simulink model "verify_Storage_Type_5_CONF_mdl"  (R2016b)
settings: Solver=ode45  StartTime=0  StopTime=6*3600  MaxStep=600  RelTol=1e-3  EnableMultiTasking=on
undefined symbols (not defined in the file or in its folder): path_carnot
libraries: carnot x20, simulink x6
settings Model: DEBUGGLOBALLEVEL=FATALLEVEL  DEBUGMAXTOTALWARNINGS=0  DEBUGMAXCONSECUTIVEWARNINGS=0  DEBUGWRITETOFILE=0  DEBUGFILENAME='error.txt'  Creator=drhf  LastModifiedBy=drhf
settings DataIOCC: SaveFormat=Array  SignalLoggingSaveFormat=ModelDataLogs
settings OptimizationCC: ExpressionDepthLimit=2147483647  LifeSpan=inf
settings DebuggingCC: UnderspecifiedInitializationDetection=Classic  MergeDetectMultiDrivingBlocksExec=none  SolverPrmCheckMsg=warning  FcnCallInpInsideContextMsg=warning  StateNameClashWarn=warning  SFUnexpectedBacktrackingDiag=warning  SFNoUnconditionalDefaultTransitionDiag=warning  SFExecutionAtInitializationDiag=none
settings HardwareCC: ProdBitPerPointer=32  ProdBitPerSizeT=32  ProdBitPerPtrDiffT=32  ProdLargestAtomicFloat=None  ProdIntDivRoundTo=Undefined  ProdEndianess=Unspecified  ProdWordSize=32  ProdHWDeviceType=32-bit Generic
settings ModelReferenceCC: PropagateSignalLabelsOutOfModel=off
settings GRTTargetCC: TargetLangStandard=C89/C90 (ANSI)  GeneratePreprocessorConditionals=Disable all  CombineOutputUpdateFcns=off  GRTInterface=on
settings ConfigComp: CovMetricSettings=dw  CovHtmlReporting=on  CovSaveCumulativeToWorkspaceVar=on  CovSaveSingleToWorkspaceVar=on  CovExternalEMLEnable=off

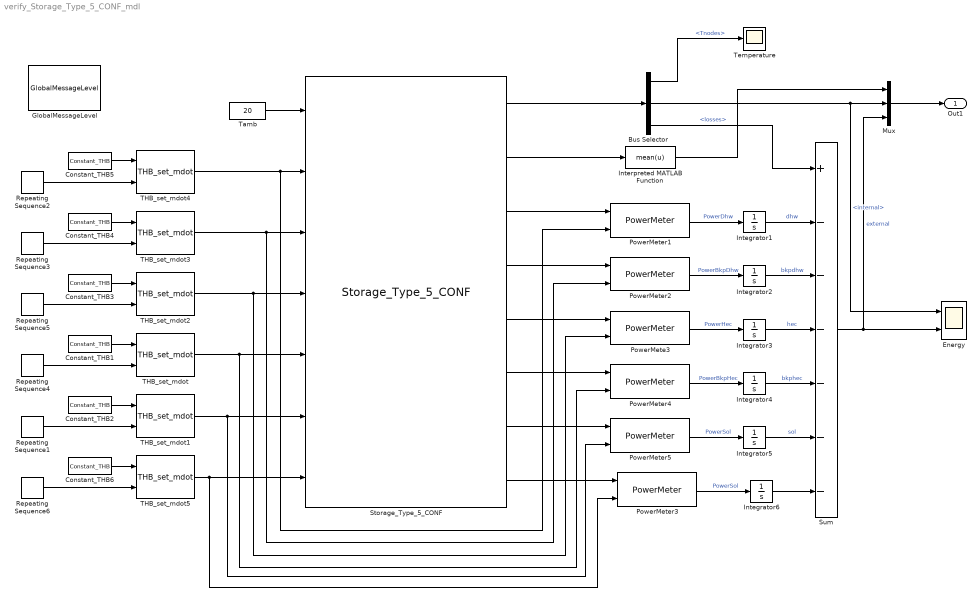
== system verify_Storage_Type_5_CONF_mdl ==
  Bus Selector : BusSelector  OutputSignals=Tnodes,energy.internal,energy.losses
  Constant_THB1 : carnot/Source/Simple/Constant_THB  t=40  mdot=100/3600  p=1e5  mID=No Pressure Drop  fluid=Water  mix=0  mix2=0  mix3=0  dia=0.02  hgt=0
  Constant_THB2 : carnot/Source/Simple/Constant_THB  t=40  mdot=100/3600  p=1e5  mID=No Pressure Drop  fluid=Water  mix=0  mix2=0  mix3=0  dia=0.02  hgt=0
  Constant_THB3 : carnot/Source/Simple/Constant_THB  t=30  mdot=100/3600  p=1e5  mID=No Pressure Drop  fluid=Water  mix=0  mix2=0  mix3=0  dia=0.02  hgt=0
  Constant_THB4 : carnot/Source/Simple/Constant_THB  t=70  mdot=100/3600  p=1e5  mID=No Pressure Drop  fluid=Water  mix=0  mix2=0  mix3=0  dia=0.02  hgt=0
  Constant_THB5 : carnot/Source/Simple/Constant_THB  t=15  mdot=0  p=1e5  mID=No Pressure Drop  fluid=Water  mix=0  mix2=0  mix3=0  dia=0.02  hgt=0
  Constant_THB6 : carnot/Source/Simple/Constant_THB  t=40  mdot=100/3600  p=1e5  mID=No Pressure Drop  fluid=Water  mix=0  mix2=0  mix3=0  dia=0.02  hgt=0
  Energy : Scope  NumInputPorts=2
  GlobalMessageLevel : carnot/Toolbox/GlobalMessageLevel  GLOBALLOCAL=global  DEBUGLEVEL=FATALLEVEL  MAXTOTALWARNINGS=0  MAXCONSECUTIVEWARNINGS=0  WRITETOFILE=0  FILENAME='error.txt'
  Integrator{1..6} (6 alike) : Integrator
  Interpreted MATLAB Function : MATLABFcn  MATLABFcn=mean(u)
  Mux : Mux  Inputs=3
  PowerMete3 : carnot/Control/PowerMeter
  PowerMeter{1..5} (5 alike) : carnot/Control/PowerMeter
  Repeating Sequence1 : simulink/Sources/Repeating Sequence  rep_seq_t=[ 0 3600 3601 7200 7201 10800]  rep_seq_y=[ 0.12 0.12 0.11 0.11 0.05 0.05]
  Repeating Sequence2 : simulink/Sources/Repeating Sequence  rep_seq_t=[ 0 3600 3601 7200 7201 10440 10441 11160]  rep_seq_y=[ 0 0 0.05 0.05 0.2 0.2 0 0]
  Repeating Sequence3 : simulink/Sources/Repeating Sequence  rep_seq_t=[ 0 3600 3601 7200 7201 10800]  rep_seq_y=[ 0 0 0.1 0.1 0.15 0.15]
  Repeating Sequence4 : simulink/Sources/Repeating Sequence  rep_seq_t=[ 0 3600 3601 7200 7201 10800]  rep_seq_y=[ 0.11 0.11 0.1 0.1 0.11 0.11]
  Repeating Sequence5 : simulink/Sources/Repeating Sequence  rep_seq_t=[ 0 3600 3601 7200 7201 10800]  rep_seq_y=[ 0.11 0.11 0.1 0.1 0.11 0.11]
  Repeating Sequence6 : simulink/Sources/Repeating Sequence  rep_seq_t=[ 0 3600 3601 7200 7201 10800]  rep_seq_y=[ 0 0 0.01 0.01 0.05 0.05]
  Storage_Type_5_CONF : carnot/Storage/Thermal/Storage_Type_5_CONF  t0=[10:5:55]  hgt=1.8108  stgtype=5  tini=[10 12.3684210526316 14.7368421052632 17.1052631578947 19.4736842105263 21.8421052631579 24.2105263157895 26.5789473684211 28.9473684210526 31.3157894736842 33.6842105263158 36.0526315789474 38.4210526315789 40.7894736842105 43.1578947368421 45.5263157894737 47.8947368421053 50.2631578947368 52.6315789473684 55]  mpts=[1 3 5 7 9 11 13 15 17 19]  PathName=fullfile(path_carnot('libsl'),'Storage','Thermal','Storage_Type_5_CONF','parameter_set')  FileName='StorageType5_800_L.mat'  userPath=off  userParam=off  uwall=1  ubot=1  utop=1  axcond=1  volume=0.8  dia=0.75  standing=standing cylinder  nodes=20  mpoints=10  Tsensor=[0.2 0.5 0.7]  pipe3inlet=1  pipe3outlet=0.6  pipe3dia=0.05  pipe1inlet=0.55  pipe1outlet=0.45  pipe1dia=0.05  hx1inlet=0.4  hx1outlet=0  hx1dia=0.03  hx1uac=200  hx1uam=0.15  hx1uat=0.6  hx1dplin=20  hx1dpqua=20  pipe2inlet=0.45  pipe2outlet=0.55  pipe2dia=0.05  hx2inlet=0  hx2outlet=1  hx2dia=0.025  hx2uac=450  hx2uam=0.4  hx2uat=0.8  hx2dplin=200  hx2dpqua=200  hx3inlet=0.9  hx3outlet=1  hx3dia=0.01  hx3uac=100  hx3uam=0  hx3uat=0  hx3dplin=10  hx3dpqua=10
  Sum : Sum  Inputs=+------
  THB_set_mdot{,1..5} (6 alike) : carnot/Source/Simple/THB_set_mdot
  Tamb : Constant  Value=20
  Temperature : Scope
  Out1 : Outport
  wires:
  Mux/1 -> Out1/1
  Tamb/1 -> Storage_Type_5_CONF/1
  Constant_THB1/1 -> THB_set_mdot/1
  THB_set_mdot/1 -> PowerMeter4/2, Storage_Type_5_CONF/5
  THB_set_mdot1/1 -> PowerMeter5/2, Storage_Type_5_CONF/6
  Constant_THB2/1 -> THB_set_mdot1/1
  Repeating Sequence4/1 -> THB_set_mdot/2
  Repeating Sequence1/1 -> THB_set_mdot1/2
  Storage_Type_5_CONF/2 -> Interpreted MATLAB Function/1
  PowerMeter1/1 -> Integrator1/1  "PowerDhw"
  PowerMeter2/1 -> Integrator2/1  "PowerBkpDhw"
  Bus Selector/1 -> Temperature/1  "<Tnodes>"
  Repeating Sequence2/1 -> THB_set_mdot4/2
  Bus Selector/2 -> Energy/1, Mux/2  "<internal>"
  Constant_THB3/1 -> THB_set_mdot2/1
  Repeating Sequence5/1 -> THB_set_mdot2/2
  THB_set_mdot2/1 -> PowerMete3/2, Storage_Type_5_CONF/4
  THB_set_mdot4/1 -> PowerMeter1/2, Storage_Type_5_CONF/2
  Constant_THB4/1 -> THB_set_mdot3/1
  Repeating Sequence3/1 -> THB_set_mdot3/2
  THB_set_mdot3/1 -> PowerMeter2/2, Storage_Type_5_CONF/3
  Storage_Type_5_CONF/1 -> Bus Selector/1
  Storage_Type_5_CONF/3 -> PowerMeter1/1
  Storage_Type_5_CONF/4 -> PowerMeter2/1
  Storage_Type_5_CONF/5 -> PowerMete3/1
  Storage_Type_5_CONF/6 -> PowerMeter4/1
  Storage_Type_5_CONF/7 -> PowerMeter5/1
  PowerMete3/1 -> Integrator3/1  "PowerHec"
  PowerMeter4/1 -> Integrator4/1  "PowerBkpHec"
  PowerMeter5/1 -> Integrator5/1  "PowerSol"
  Integrator1/1 -> Sum/2  "dhw"
  Integrator2/1 -> Sum/3  "bkpdhw"
  Integrator3/1 -> Sum/4  "hec"
  Integrator4/1 -> Sum/5  "bkphec"
  Integrator5/1 -> Sum/6  "sol"
  Sum/1 -> Energy/2, Mux/3  "external"
  Interpreted MATLAB Function/1 -> Mux/1
  Bus Selector/3 -> Sum/1  "<losses>"
  Constant_THB5/1 -> THB_set_mdot4/1
  PowerMeter3/1 -> Integrator6/1  "PowerSol"
  Integrator6/1 -> Sum/7
  Storage_Type_5_CONF/8 -> PowerMeter3/1
  Constant_THB6/1 -> THB_set_mdot5/1
  Repeating Sequence6/1 -> THB_set_mdot5/2
  THB_set_mdot5/1 -> PowerMeter3/2, Storage_Type_5_CONF/7
